simulink model "CarControl"  (R2016a)
settings: Solver=FixedStepDiscrete  StartTime=0.0  StopTime=15  FixedStep=0.01  RelTol=1e-3
undefined symbols (not defined in the file or in its folder): DiscIntNeverNeededParam
libraries: simulink x5, aerolibanimutils x1
settings Model: Creator=uos  LastModifiedBy=uos
settings GRTTargetCC: GeneratePreprocessorConditionals=Use local settings

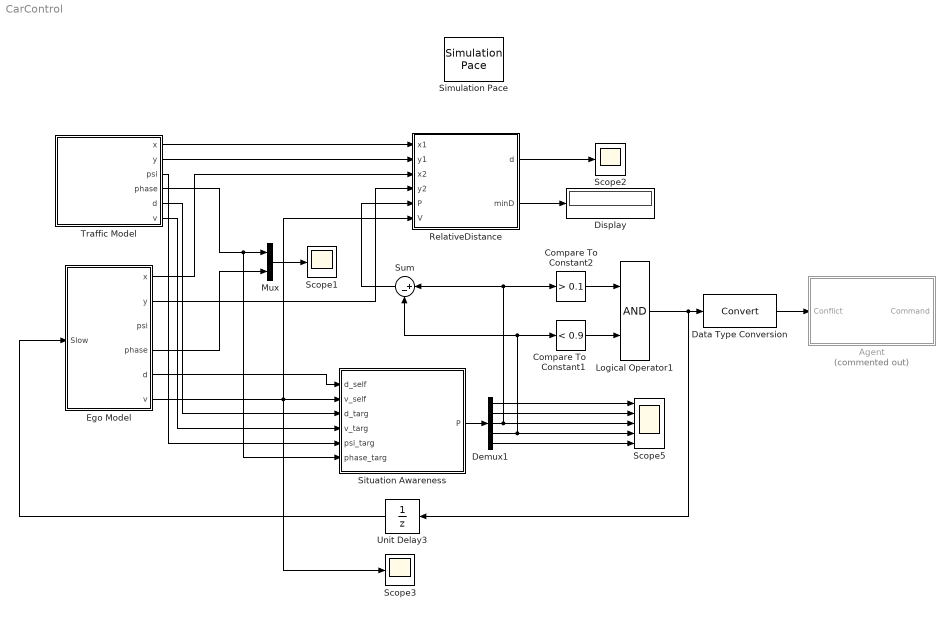
== system CarControl ==
  Agent : Subsystem  Commented=on
  Compare To Constant1 : simulink/Logic and Bit Operations/Compare To Constant  relop=<  const=0.9  OutDataTypeStr=boolean
  Compare To Constant2 : simulink/Logic and Bit Operations/Compare To Constant  relop=>  const=0.1  OutDataTypeStr=boolean
  Data Type Conversion : DataTypeConversion
  Demux1 : Demux  Outputs=5
  Display : Display
  Ego Model : Subsystem
  Logical Operator1 : Logic  AllPortsSameDT=off  OutDataTypeStr=boolean
  Mux : Mux  Inputs=2
  RelativeDistance : Subsystem
  Scope1 : Scope
  Scope2 : Scope
  Scope3 : Scope
  Scope5 : Scope  NumInputPorts=5
  Simulation Pace : aerolibanimutils/Simulation Pace  SimulationPace=1  SleepMode=MATLAB Thread  OutputPaceError=off  SampleTime=0.01
  Situation Awareness : MATLAB Function  TreatAsAtomicUnit=on
  Sum : Sum  Inputs=|+-
  Traffic Model : Subsystem
  Unit Delay3 : UnitDelay  SampleTime=-1
  wires:
  Data Type Conversion/1 -> Agent/1(Conflict)
  Traffic Model/4(phase) -> Situation Awareness/6(phase_targ), Mux/1
  Ego Model/4(phase) -> Mux/2
  Mux/1 -> Scope1/1
  Traffic Model/1(x) -> RelativeDistance/1(x1)
  Traffic Model/2(y) -> RelativeDistance/2(y1)
  Ego Model/1(x) -> RelativeDistance/3(x2)
  Ego Model/2(y) -> RelativeDistance/4(y2)
  RelativeDistance/1(d) -> Scope2/1
  Ego Model/5(d) -> Situation Awareness/1(d_self)
  Ego Model/6(v) -> RelativeDistance/6(V), Scope3/1, Situation Awareness/2(v_self)
  Traffic Model/5(d) -> Situation Awareness/3(d_targ)
  Traffic Model/6(v) -> Situation Awareness/4(v_targ)
  Situation Awareness/1(P) -> Demux1/1
  Logical Operator1/1 -> Unit Delay3/1, Data Type Conversion/1
  Unit Delay3/1 -> Ego Model/1(Slow)
  Compare To Constant1/1 -> Logical Operator1/2
  Compare To Constant2/1 -> Logical Operator1/1
  Demux1/2 -> Scope5/2
  Demux1/1 -> Scope5/1
  Demux1/3 -> Scope5/3, Sum/1, Compare To Constant2/1
  Demux1/4 -> Scope5/4, Sum/2, Compare To Constant1/1
  Demux1/5 -> Scope5/5
  Traffic Model/3(psi) -> Situation Awareness/5(psi_targ)
  Sum/1 -> RelativeDistance/5(P)
  RelativeDistance/2(minD) -> Display/1

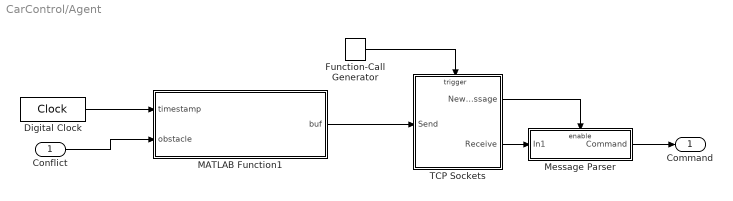
== system CarControl/Agent ==
  Conflict : Inport
  Digital Clock : DigitalClock  SampleTime=0.1
  Function-Call Generator : simulink/Ports & Subsystems/Function-Call Generator  sample_time=0.1  numberOfIterations=1
  MATLAB Function1 : MATLAB Function  TreatAsAtomicUnit=on
  Message Parser : Subsystem  TreatAsAtomicUnit=on
  TCP Sockets : Subsystem  TreatAsAtomicUnit=on
  Command : Outport
  wires:
  MATLAB Function1/1(buf) -> TCP Sockets/1(Send)
  Function-Call Generator/1 -> TCP Sockets/Trigger
  TCP Sockets/2(Receive) -> Message Parser/1(In1)
  TCP Sockets/1(NewMessage) -> Message Parser/Enable
  Digital Clock/1 -> MATLAB Function1/1(timestamp)
  Conflict/1 -> MATLAB Function1/2(obstacle)
  Message Parser/1(Command) -> Command/1

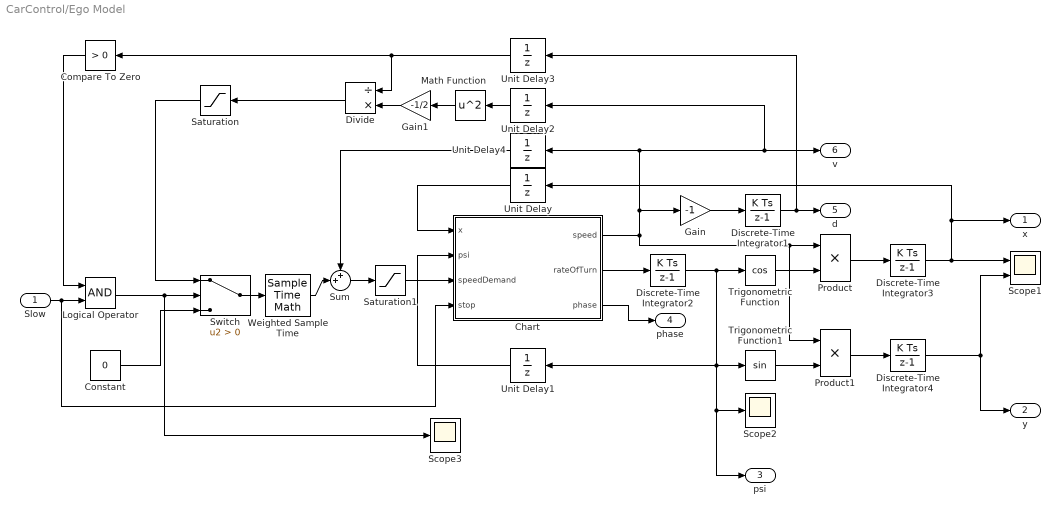
== system CarControl/Ego Model ==
  Slow : Inport
  Chart : Stateflow chart  TreatAsAtomicUnit=on
  Compare To Zero : simulink/Logic and Bit Operations/Compare To Zero  relop=>  OutDataTypeStr=boolean
  Constant : Constant  Value=0
  Discrete-Time Integrator1 : DiscreteIntegrator  gainval=1  InitialCondition=85  InitialConditionSetting=State (most efficient)  SampleTime=-1  ICPrevOutput=DiscIntNeverNeededParam  ICPrevScaledInput=DiscIntNeverNeededParam
  Discrete-Time Integrator2 : DiscreteIntegrator  InitialConditionSetting=State (most efficient)  SampleTime=-1  ICPrevOutput=DiscIntNeverNeededParam  ICPrevScaledInput=DiscIntNeverNeededParam
  Discrete-Time Integrator3 : DiscreteIntegrator  InitialCondition=-100  InitialConditionSetting=State (most efficient)  SampleTime=-1  ICPrevOutput=DiscIntNeverNeededParam  ICPrevScaledInput=DiscIntNeverNeededParam
  Discrete-Time Integrator4 : DiscreteIntegrator  InitialCondition=2  InitialConditionSetting=State (most efficient)  SampleTime=-1  ICPrevOutput=DiscIntNeverNeededParam  ICPrevScaledInput=DiscIntNeverNeededParam
  Divide : Product  Inputs=/*
  Gain : Gain  Gain=-1
  Gain1 : Gain  Gain=-1/2
  Logical Operator : Logic  AllPortsSameDT=off  OutDataTypeStr=boolean
  Math Function : Math  Operator=square  SaturateOnIntegerOverflow=on
  Product : Product
  Product1 : Product
  Saturation : Saturate  UpperLimit=3  LowerLimit=-3
  Saturation1 : Saturate  UpperLimit=Inf  LowerLimit=0
  Scope1 : Scope  NumInputPorts=2
  Scope2 : Scope
  Scope3 : Scope
  Sum : Sum  Inputs=++|
  Switch : Switch  Criteria=u2 > Threshold
  Trigonometric Function : Trigonometry  Operator=cos
  Trigonometric Function1 : Trigonometry
  Unit Delay{,1..3} (4 alike) : UnitDelay  SampleTime=-1
  Unit Delay4 : UnitDelay  InitialCondition=15  SampleTime=-1
  Weighted Sample Time : SampleTimeMath  TsampMathOp=*
  x : Outport
  y : Outport  Port=2
  psi : Outport  Port=3
  phase : Outport  Port=4
  d : Outport  Port=5
  v : Outport  Port=6
  wires:
  Chart/2(rateOfTurn) -> Discrete-Time Integrator2/1
  Discrete-Time Integrator3/1 -> Scope1/1, Unit Delay/1, x/1
  Unit Delay/1 -> Chart/1(x)
  Discrete-Time Integrator4/1 -> Scope1/2, y/1
  Unit Delay1/1 -> Chart/2(psi)
  Product/1 -> Discrete-Time Integrator3/1
  Product1/1 -> Discrete-Time Integrator4/1
  Trigonometric Function/1 -> Product/2
  Trigonometric Function1/1 -> Product1/2
  Discrete-Time Integrator2/1 -> Trigonometric Function1/1, Unit Delay1/1, Scope2/1, psi/1, Trigonometric Function/1
  Chart/3(phase) -> phase/1
  Discrete-Time Integrator1/1 -> Unit Delay3/1, d/1
  Chart/1(speed) -> Product/1, Product1/1, Unit Delay2/1, v/1, Unit Delay4/1, Gain/1
  Gain/1 -> Discrete-Time Integrator1/1
  Unit Delay2/1 -> Math Function/1
  Math Function/1 -> Gain1/1
  Gain1/1 -> Divide/2
  Unit Delay3/1 -> Compare To Zero/1, Divide/1
  Switch/1 -> Weighted Sample Time/1
  Weighted Sample Time/1 -> Sum/2
  Sum/1 -> Saturation1/1
  Unit Delay4/1 -> Sum/1
  Slow/1 -> Chart/4(stop), Logical Operator/2
  Compare To Zero/1 -> Logical Operator/1
  Logical Operator/1 -> Scope3/1, Switch/2
  Divide/1 -> Saturation/1
  Constant/1 -> Switch/3
  Saturation/1 -> Switch/1
  Saturation1/1 -> Chart/3(speedDemand)

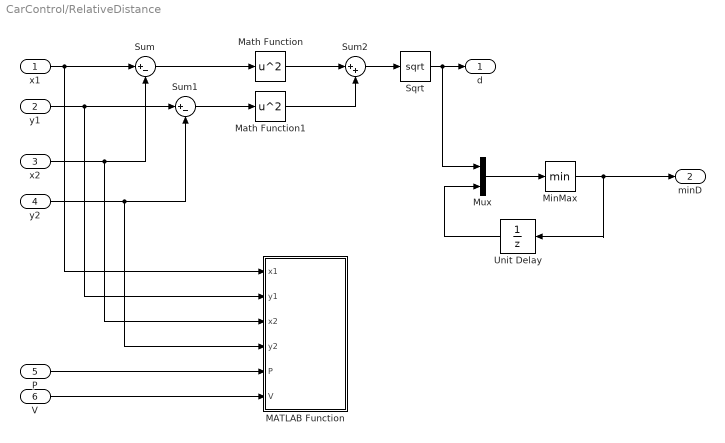
== system CarControl/RelativeDistance ==
  x1 : Inport
  y1 : Inport  Port=2
  x2 : Inport  Port=3
  y2 : Inport  Port=4
  P : Inport  Port=5
  V : Inport  Port=6
  MATLAB Function : MATLAB Function  TreatAsAtomicUnit=on
  Math Function : Math  Operator=square  SaturateOnIntegerOverflow=on
  Math Function1 : Math  Operator=square  SaturateOnIntegerOverflow=on
  MinMax : MinMax
  Mux : Mux  Inputs=2
  Sqrt : Sqrt  SaturateOnIntegerOverflow=on
  Sum : Sum  Inputs=|+-
  Sum1 : Sum  Inputs=|+-
  Sum2 : Sum  Inputs=|++
  Unit Delay : UnitDelay  InitialCondition=Inf  SampleTime=-1
  d : Outport
  minD : Outport  Port=2
  wires:
  x1/1 -> MATLAB Function/1(x1), Sum/1
  x2/1 -> MATLAB Function/3(x2), Sum/2
  y1/1 -> MATLAB Function/2(y1), Sum1/1
  y2/1 -> MATLAB Function/4(y2), Sum1/2
  Sum/1 -> Math Function/1
  Sum1/1 -> Math Function1/1
  Math Function/1 -> Sum2/1
  Math Function1/1 -> Sum2/2
  Sum2/1 -> Sqrt/1
  Sqrt/1 -> Mux/1, d/1
  P/1 -> MATLAB Function/5(P)
  V/1 -> MATLAB Function/6(V)
  Mux/1 -> MinMax/1
  MinMax/1 -> Unit Delay/1, minD/1
  Unit Delay/1 -> Mux/2

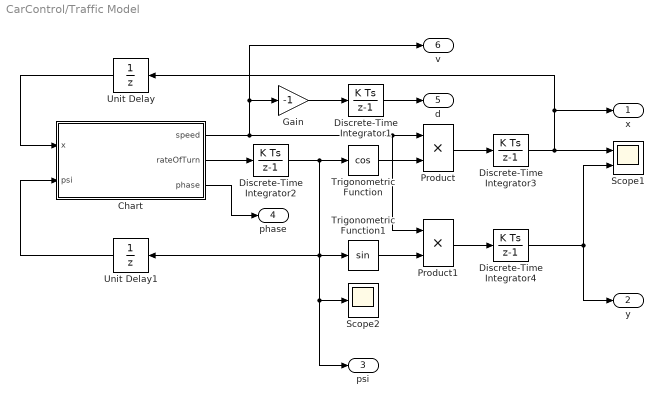
== system CarControl/Traffic Model ==
  Chart : Stateflow chart  TreatAsAtomicUnit=on
  Discrete-Time Integrator1 : DiscreteIntegrator  InitialCondition=30  InitialConditionSetting=State (most efficient)  SampleTime=-1  ICPrevOutput=DiscIntNeverNeededParam  ICPrevScaledInput=DiscIntNeverNeededParam
  Discrete-Time Integrator2 : DiscreteIntegrator  InitialCondition=pi  InitialConditionSetting=State (most efficient)  SampleTime=-1  ICPrevOutput=DiscIntNeverNeededParam  ICPrevScaledInput=DiscIntNeverNeededParam
  Discrete-Time Integrator3 : DiscreteIntegrator  InitialCondition=45  InitialConditionSetting=State (most efficient)  SampleTime=-1  ICPrevOutput=DiscIntNeverNeededParam  ICPrevScaledInput=DiscIntNeverNeededParam
  Discrete-Time Integrator4 : DiscreteIntegrator  InitialCondition=-2  InitialConditionSetting=State (most efficient)  SampleTime=-1  ICPrevOutput=DiscIntNeverNeededParam  ICPrevScaledInput=DiscIntNeverNeededParam
  Gain : Gain  Gain=-1
  Product : Product
  Product1 : Product
  Scope1 : Scope  NumInputPorts=2
  Scope2 : Scope
  Trigonometric Function : Trigonometry  Operator=cos
  Trigonometric Function1 : Trigonometry
  Unit Delay : UnitDelay  SampleTime=-1
  Unit Delay1 : UnitDelay  SampleTime=-1
  x : Outport
  y : Outport  Port=2
  psi : Outport  Port=3
  phase : Outport  Port=4
  d : Outport  Port=5
  v : Outport  Port=6
  wires:
  Discrete-Time Integrator2/1 -> Trigonometric Function/1, psi/1, Scope2/1, Unit Delay1/1, Trigonometric Function1/1
  Trigonometric Function1/1 -> Product1/2
  Trigonometric Function/1 -> Product/2
  Product1/1 -> Discrete-Time Integrator4/1
  Product/1 -> Discrete-Time Integrator3/1
  Unit Delay1/1 -> Chart/2(psi)
  Discrete-Time Integrator4/1 -> y/1, Scope1/2
  Unit Delay/1 -> Chart/1(x)
  Discrete-Time Integrator3/1 -> x/1, Unit Delay/1, Scope1/1
  Chart/2(rateOfTurn) -> Discrete-Time Integrator2/1
  Chart/3(phase) -> phase/1
  Chart/1(speed) -> Product1/1, Product/1, v/1, Gain/1
  Discrete-Time Integrator1/1 -> d/1
  Gain/1 -> Discrete-Time Integrator1/1

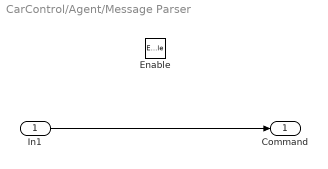
== system CarControl/Agent/Message Parser ==
  In1 : Inport
  Enable : EnablePort
  Command : Outport
  wires:
  In1/1 -> Command/1

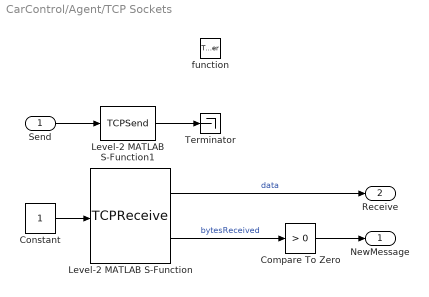
== system CarControl/Agent/TCP Sockets ==
  Send : Inport
  function : TriggerPort  TriggerType=function-call  VariantControl=Variant
  Compare To Zero : simulink/Logic and Bit Operations/Compare To Zero  relop=>  OutDataTypeStr=boolean
  Constant : Constant
  Level-2 MATLAB S-Function : M-S-Function  Priority=2  FunctionName=TCPReceive  Parameters='127.0.0.1',18000,[1 1],1,0.5,-1,'int32','LittleEndian'
  Level-2 MATLAB S-Function1 : M-S-Function  Priority=1  FunctionName=TCPSend  Parameters='127.0.0.1',17000,0,0.5,'LittleEndian'
  Terminator : Terminator
  NewMessage : Outport
  Receive : Outport  Port=2
  wires:
  Level-2 MATLAB S-Function/1 -> Receive/1  "data"
  Send/1 -> Level-2 MATLAB S-Function1/1
  Level-2 MATLAB S-Function/2 -> Compare To Zero/1  "bytesReceived"
  Compare To Zero/1 -> NewMessage/1
  Constant/1 -> Level-2 MATLAB S-Function/1
  Level-2 MATLAB S-Function1/1 -> Terminator/1

== stateflow chart CarControl/Traffic Model/Chart ==
  state ApproachRoundabout
    en:speed = 15;
    en:rateOfTurn = 0;
    en: phase = 0;
  state ExitRoundabout
    en:rateOfTurn = pi/4;
    en:speed = 4*rateOfTurn;
    en: phase = phase + 1;
  state EnterRoundabout
    en:rateOfTurn = pi/4;
    en:speed = 2.5*rateOfTurn;
    en: phase = phase + 1;
  state OnRoundabout
    en: rateOfTurn = -rateOfTurn;
    en: speed = -12.9*rateOfTurn;
    en: phase = phase + 1;
  state OffRoundabout
    en:speed = 15;
    en:rateOfTurn = 0;
    en: phase = phase + 1;
  (default) -> ApproachRoundabout
  OnRoundabout -> ExitRoundabout : [psi<=deg2rad(22)]
  EnterRoundabout -> OnRoundabout : [psi>=deg2rad(255)]
  ApproachRoundabout -> EnterRoundabout : [x<=15]
  ExitRoundabout -> OffRoundabout : [psi > pi/2]
  data: x input; speed output; rateOfTurn output; psi input; phase output

== matlab function CarControl/RelativeDistance/MATLAB Function ==
  data: x1 input; y1 input; x2 input; y2 input; P input; V input
function fcn(x1, y1, x2, y2, P, V)
%#codegen

coder.extrinsic('plotProgress')
persistent start
if isempty(start)
    close all
    start = 1;
end
plotProgress(x1, y1, x2, y2, P, V);

== stateflow chart CarControl/Ego Model/Chart ==
  state ExitRoundabout
    en:rateOfTurn = pi/4;
    en:speed = 4*rateOfTurn;
    en: phase = phase + 1;
  state ApproachRoundabout
    en:speed = 15;
    en:rateOfTurn = 0;
    en: phase = 0;
    du: speed = speedDemand;
  state EnterRoundabout
    en:rateOfTurn = pi/4;
    en:speed = 2.5*rateOfTurn;
    en: phase = phase + 1;
  state OnRoundabout
    en: rateOfTurn = -rateOfTurn;
    en: speed = -12.9*rateOfTurn;
    en: phase = phase + 1;
  state OffRoundabout
    en:speed = 15;
    en:rateOfTurn = 0;
    en: phase = phase + 1;
  (default) -> ApproachRoundabout
  OnRoundabout -> ExitRoundabout : [psi<=deg2rad(-90+22)]
  EnterRoundabout -> OnRoundabout : [psi>=deg2rad(75)]
  ApproachRoundabout -> EnterRoundabout : [x>=-15 && ~stop]
  ExitRoundabout -> OffRoundabout : [psi > 0]
  data: x input; speed output; rateOfTurn output; psi input; phase output; speedDemand input; stop input

== matlab function CarControl/Situation Awareness ==
  data: d_self input; P output; v_self input; d_targ input; v_targ input; psi_targ input; phase_targ input
function P  = fcn(d_self, v_self, d_targ, v_targ, psi_targ, phase_targ)
%#codegen
persistent t_bar;
if isempty(t_bar)
    t_bar = [0 0 0 0 0];
end
t_barO = t_bar;
t_barSelf = [0 0 0 0 0];
t_var = [0 0 0 0 0];
P = [0 0 0 0 0]';

% Only concerned with projection until we entre roundabout
if v_self > 0 && d_self < -1
    return
end

% Enter Roundabout
t_bar(1) = d_targ/v_targ;
t_var(1) = sqrt((1*d_targ/v_targ^2)^2 + (0.25/v_targ)^2);

if phase_targ < 1
    % On roundabout
    t_bar(2) = deg2rad(75)/(pi/4);
    t_var(2) = ((pi/2/45)*(deg2rad(75)))/(pi/4)^2;
else
    t_bar(1) = 0;
    t_var(1) = 0;
    % On roundabout
    t_bar(2) = (deg2rad(75) - psi_targ + pi)/(pi/4);
    t_var(2) = ((pi/2/45)*(deg2rad(75) - psi_targ + pi))/(pi/4)^2;
end

if phase_targ < 2
    % On roundabout 2
    t_bar(3) = deg2rad(75)/(pi/4);
    t_var(3) = ((pi/2/45)*(deg2rad(75)))/(pi/4)^2;
else
    t_bar(2) = 0;
    t_var(2) = 0;
    t_bar(3) = (deg2rad(75) + psi_targ - pi - deg2rad(75))/(pi/4);
    t_var(3) = ((pi/2/45)*(deg2rad(75) + psi_targ - pi - deg2rad(75)))/(pi/4)^2;
end
% r = v_targ/(pi/4);
% ang = abs(d_targ)/r;

% Exit roundabout
t_bar(4) = (pi/2 + deg2rad(68))/(pi/4);
t_var(4) = ((pi/2/45)*(pi/2 + deg2rad(68)))/(pi/4)^2;

% Off roundabout
t_bar(5) = (deg2rad(68))/(pi/4);
t_var(5) = ((pi/2/45)*(deg2rad(68)))/(pi/4)^2;


t_self = d_self/v_self; t_barSelf(1) = t_self;

P(1) = normcdf(t_self,t_bar(1),t_var(1));

%t_self = t_self + deg2rad(75)/(pi/4); t_barSelf(2) = t_self;
P(2) = normcdf(t_self,sum(t_bar(1:2)),sqrt(sum(t_var(1:2).^2)));

%t_self = t_self + deg2rad(75-25+90)/(pi/4); t_barSelf(3) = t_self;
P(3) = normcdf(t_self,sum(t_bar(1:3)),sqrt(sum(t_var(1:3).^2)));

%t_self = t_self + deg2rad(68)/(pi/4); t_barSelf(4) = t_self;
P(4) = normcdf(t_self,sum(t_bar(1:4)),sqrt(sum(t_var(1:4).^2)));


t_barO = cumsum(t_bar);

== matlab function CarControl/Agent/MATLAB Function1 ==
  data: buf output; timestamp input double; obstacle input double
function buf  = fcn(timestamp, obstacle)
%#codegen

buf = zeros(4*8,1,'uint8');

n = 0;

buf(8*n + (1:8)) = typecast(timestamp,'uint8'); n = n + 1;
buf(8*n + (1:8)) = typecast(obstacle,'uint8'); n = n + 1;
buf(8*n + (1:8)) = typecast(obstacle,'uint8'); n = n + 1;
buf(8*n + (1:8)) = typecast(0,'uint8'); n = n + 1;
